simulink library "CreateSdat"  (R2018b)
settings: Solver=ode45  StartTime=0.0  StopTime=10.0  RelTol=1e-3  EnableMultiTasking=on
settings Model: Creator=drhf  LastModifiedBy=drhf
settings DataIOCC: LimitDataPoints=on  SaveFormat=Array  SignalLoggingSaveFormat=ModelDataLogs
settings OptimizationCC: ExpressionDepthLimit=2147483647  LifeSpan=inf
settings DebuggingCC: UnderspecifiedInitializationDetection=Classic  MergeDetectMultiDrivingBlocksExec=none  SolverPrmCheckMsg=warning  FcnCallInpInsideContextMsg=warning  StateNameClashWarn=warning  SFUnexpectedBacktrackingDiag=warning  SFNoUnconditionalDefaultTransitionDiag=warning  SFExecutionAtInitializationDiag=none
settings HardwareCC: ProdBitPerPointer=32  ProdBitPerSizeT=32  ProdBitPerPtrDiffT=32  ProdLargestAtomicFloat=None  ProdIntDivRoundTo=Undefined  ProdEndianess=Unspecified  ProdWordSize=32  ProdHWDeviceType=32-bit Generic
settings ModelReferenceCC: PropagateSignalLabelsOutOfModel=off
settings SFSimCC: SimUseLocalCustomCode=off
settings RTWCC: RTWUseLocalCustomCode=off
settings CodeAppCC: StateflowObjectComments=on
settings GRTTargetCC: TargetLangStandard=C89/C90 (ANSI)  GeneratePreprocessorConditionals=Disable all  CombineOutputUpdateFcns=off  GRTInterface=on
settings ConfigComp: CovMetricSettings=dw  CovHtmlReporting=on  CovSaveCumulativeToWorkspaceVar=on  CovSaveSingleToWorkspaceVar=on  CovExternalEMLEnable=off

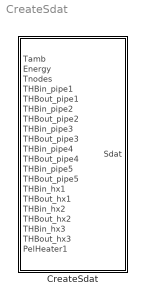
== system CreateSdat ==
  CreateSdat : Subsystem  mask(CreateSdat){volume=0.5, stgtype=1}
      mask prompts: volume "Volume of storage in m³"; stgtype "Storage Type (0..5)"
      mask help: Create the Sdat structure of the storage (Storage_Type_N). All relevant informations for further evaluation of the storage are combined in this structure. The parameter volume in the storage mask should be promoted from this block.
      mask init:
      | if isempty(volume)||~isnumeric(volume)
      |    volume = 0.1; 
      | end
      | if isempty(stgtype)||~isnumeric(stgtype)
      |    stgtype = 1; 
      | end
      mask Help: web(fullfile(path_carnot('help'),'CreateSdat.html'),'-helpbrowser')
      mask TypeOptions volume: Volume/Value
      mask TypeOptions stgtype: StgType/Value

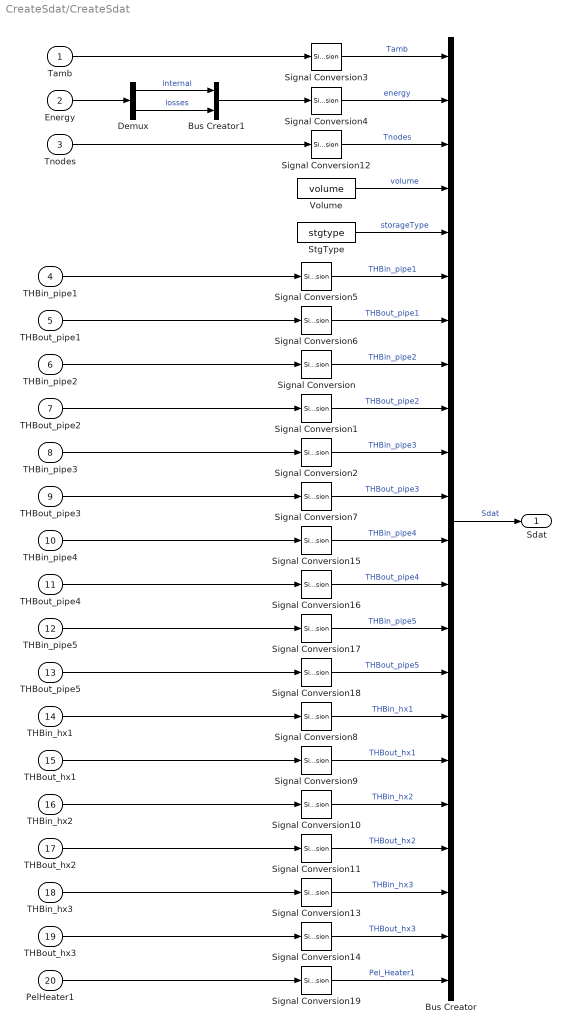
== system CreateSdat/CreateSdat ==
  Tamb : Inport
  Energy : Inport  Port=2
  Tnodes : Inport  Port=3
  THBin_pipe1 : Inport  Port=4
  THBout_pipe1 : Inport  Port=5
  THBin_pipe2 : Inport  Port=6
  THBout_pipe2 : Inport  Port=7
  THBin_pipe3 : Inport  Port=8
  THBout_pipe3 : Inport  Port=9
  THBin_pipe4 : Inport  Port=10
  THBout_pipe4 : Inport  Port=11
  THBin_pipe5 : Inport  Port=12
  THBout_pipe5 : Inport  Port=13
  THBin_hx1 : Inport  Port=14
  THBout_hx1 : Inport  Port=15
  THBin_hx2 : Inport  Port=16
  THBout_hx2 : Inport  Port=17
  THBin_hx3 : Inport  Port=18
  THBout_hx3 : Inport  Port=19
  PelHeater1 : Inport  Port=20
  Bus Creator : BusCreator  Inputs=22
  Bus Creator1 : BusCreator  Inputs=2
  Demux : Demux  Outputs=2
  Signal Conversion{,1..19} (20 alike) : SignalConversion  OverrideOpt=off
  StgType : Constant  Value=stgtype
  Volume : Constant  Value=volume
  Sdat : Outport
  wires:
  Signal Conversion19/1 -> Bus Creator/22  "Pel_Heater1"
  PelHeater1/1 -> Signal Conversion19/1
  Signal Conversion17/1 -> Bus Creator/14  "THBin_pipe5"
  THBin_pipe5/1 -> Signal Conversion17/1
  THBout_pipe5/1 -> Signal Conversion18/1
  Signal Conversion18/1 -> Bus Creator/15  "THBout_pipe5"
  Signal Conversion16/1 -> Bus Creator/13  "THBout_pipe4"
  THBout_pipe4/1 -> Signal Conversion16/1
  THBin_pipe4/1 -> Signal Conversion15/1
  Signal Conversion15/1 -> Bus Creator/12  "THBin_pipe4"
  StgType/1 -> Bus Creator/5  "storageType"
  Signal Conversion14/1 -> Bus Creator/21  "THBout_hx3"
  THBout_hx3/1 -> Signal Conversion14/1
  THBin_hx3/1 -> Signal Conversion13/1
  Signal Conversion13/1 -> Bus Creator/20  "THBin_hx3"
  Signal Conversion11/1 -> Bus Creator/19  "THBout_hx2"
  Signal Conversion2/1 -> Bus Creator/10  "THBin_pipe3"
  Signal Conversion/1 -> Bus Creator/8  "THBin_pipe2"
  Signal Conversion1/1 -> Bus Creator/9  "THBout_pipe2"
  THBout_pipe1/1 -> Signal Conversion6/1
  THBout_hx2/1 -> Signal Conversion11/1
  THBin_pipe1/1 -> Signal Conversion5/1
  Bus Creator/1 -> Sdat/1  "Sdat"
  THBin_hx2/1 -> Signal Conversion10/1
  THBout_hx1/1 -> Signal Conversion9/1
  THBin_hx1/1 -> Signal Conversion8/1
  Signal Conversion12/1 -> Bus Creator/3  "Tnodes"
  Signal Conversion6/1 -> Bus Creator/7  "THBout_pipe1"
  THBout_pipe2/1 -> Signal Conversion1/1
  Signal Conversion9/1 -> Bus Creator/17  "THBout_hx1"
  Signal Conversion4/1 -> Bus Creator/2  "energy"
  Signal Conversion8/1 -> Bus Creator/16  "THBin_hx1"
  Tamb/1 -> Signal Conversion3/1
  THBin_pipe3/1 -> Signal Conversion2/1
  Tnodes/1 -> Signal Conversion12/1
  Signal Conversion10/1 -> Bus Creator/18  "THBin_hx2"
  THBout_pipe3/1 -> Signal Conversion7/1
  Signal Conversion7/1 -> Bus Creator/11  "THBout_pipe3"
  Signal Conversion5/1 -> Bus Creator/6  "THBin_pipe1"
  THBin_pipe2/1 -> Signal Conversion/1
  Signal Conversion3/1 -> Bus Creator/1  "Tamb"
  Demux/2 -> Bus Creator1/2  "losses"
  Demux/1 -> Bus Creator1/1  "internal"
  Energy/1 -> Demux/1
  Bus Creator1/1 -> Signal Conversion4/1
  Volume/1 -> Bus Creator/4  "volume"
